simulink model "Davinci_Simul_ValidationJ"  (R2023a)
settings: Solver=VariableStepAuto  StartTime=0.0  StopTime=10.0  MaxStep=1e-5  RelTol=1e-3
libraries: DaVinci_LibJ x1
settings Model: Creator=ASUS  LastModifiedBy=afons

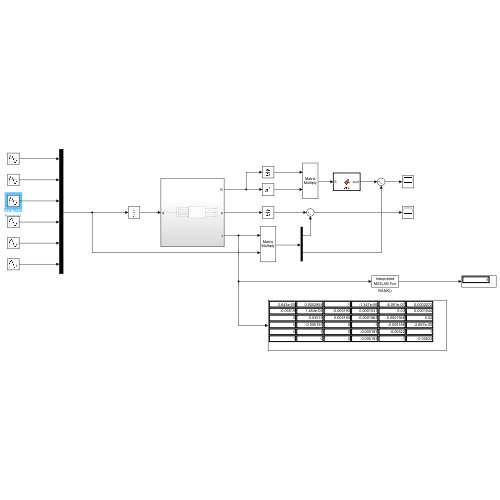
[thumbnail: Simulink's stored preview of the top-level diagram]
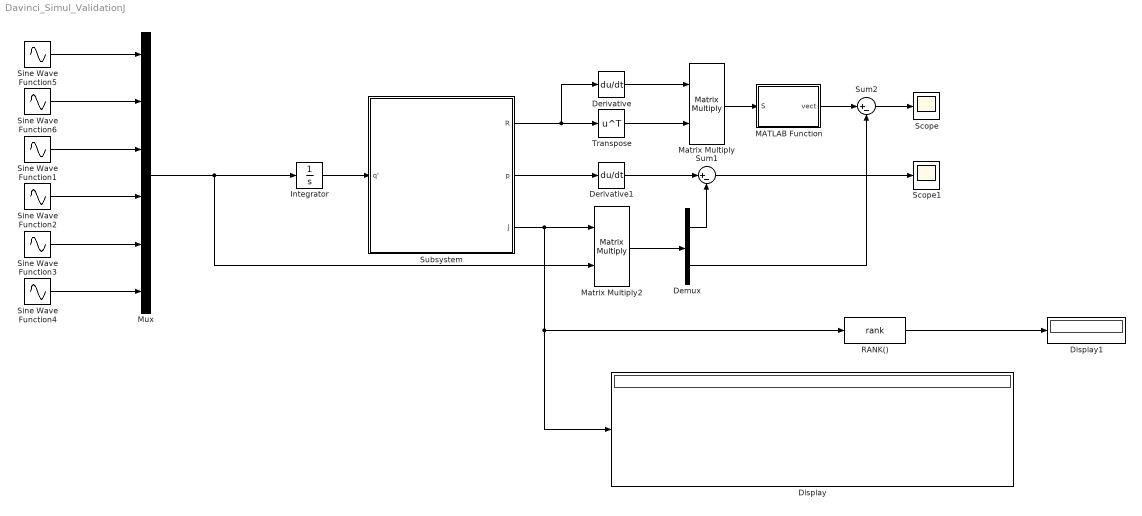
== system Davinci_Simul_ValidationJ ==
  Demux : Demux  Outputs=2
  Derivative : Derivative
  Derivative1 : Derivative
  Display : Display
  Display1 : Display
  Integrator : Integrator
  MATLAB Function : MATLAB Function  TreatAsAtomicUnit=on
  Matrix Multiply : Product  Multiplication=Matrix(*)
  Matrix Multiply2 : Product  Multiplication=Matrix(*)
  Mux : Mux  Inputs=6
  RANK() : MATLABFcn  MATLABFcn=rank
  Scope : Scope
  Scope1 : Scope
  Sine Wave Function1 : Sin  SampleTime=0  VectorParams1D=off
  Sine Wave Function{2..6} (5 alike) : Sin  SampleTime=0
  Subsystem : Subsystem
  Sum1 : Sum  Inputs=|+-
  Sum2 : Sum  Inputs=|+-
  Transpose : Math  Operator=transpose
  wires:
  Subsystem/2(p) -> Derivative1/1
  Derivative1/1 -> Sum1/1
  Derivative/1 -> Matrix Multiply/1
  Subsystem/1(R) -> Derivative/1, Transpose/1
  Transpose/1 -> Matrix Multiply/2
  Subsystem/3(J) -> RANK()/1, Display/1, Matrix Multiply2/1
  Matrix Multiply2/1 -> Demux/1
  Demux/2 -> Sum2/2
  MATLAB Function/1(vect) -> Sum2/1
  Demux/1 -> Sum1/2
  Sum1/1 -> Scope1/1
  Sum2/1 -> Scope/1
  Matrix Multiply/1 -> MATLAB Function/1(S)
  Sine Wave Function5/1 -> Mux/1
  Sine Wave Function6/1 -> Mux/2
  Sine Wave Function1/1 -> Mux/3
  Sine Wave Function2/1 -> Mux/4
  Sine Wave Function3/1 -> Mux/5
  Sine Wave Function4/1 -> Mux/6
  Mux/1 -> Matrix Multiply2/2, Integrator/1
  Integrator/1 -> Subsystem/1(q')
  RANK()/1 -> Display1/1

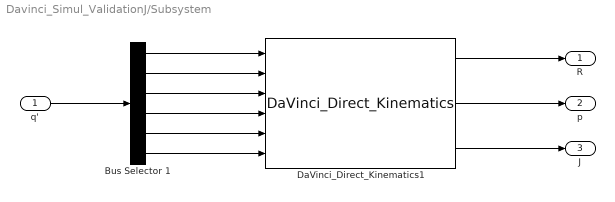
== system Davinci_Simul_ValidationJ/Subsystem ==
  q' : Inport
  Bus Selector 1 : Demux  Outputs=6
  DaVinci_Direct_Kinematics1 : DaVinci_LibJ/DaVinci_Direct_Kinematics  SystemSampleTime=-1  VariantActivationTime=update diagram  Latency=0  AutoFrameSizeCalculation=off
      settings: LibrarySourceBlock=|
      | simulink/User-Defined
      | Functions/MATLAB Function
  R : Outport
  p : Outport  Port=2
  J : Outport  Port=3
  wires:
  Bus Selector 1/2 -> DaVinci_Direct_Kinematics1/2
  Bus Selector 1/6 -> DaVinci_Direct_Kinematics1/6
  Bus Selector 1/3 -> DaVinci_Direct_Kinematics1/3
  Bus Selector 1/1 -> DaVinci_Direct_Kinematics1/1
  Bus Selector 1/5 -> DaVinci_Direct_Kinematics1/5
  Bus Selector 1/4 -> DaVinci_Direct_Kinematics1/4
  DaVinci_Direct_Kinematics1/1 -> R/1
  q'/1 -> Bus Selector 1/1
  DaVinci_Direct_Kinematics1/2 -> p/1
  DaVinci_Direct_Kinematics1/3 -> J/1

== matlab function Davinci_Simul_ValidationJ/MATLAB Function ==
  data: S input; vect output
function vect  = vec(S)
% recebe a matrix anti-inversa que resulta do produto de R* com Rt
vect = [S(3,2);S(1,3);S(2,1)];
end
